simulink model ""  (R2025a)
settings: Solver=FixedStepDiscrete  StartTime=0.0  StopTime=inf  FixedStep=0.001  RelTol=1e-3  EnableMultiTasking=on
PreLoadFcn:
  | frs = FrankaRobotSettings;
libraries: franka_simulink x1
settings Model: SimulationMode=external  ExtModeTrigDuration=10000  Creator=vasi_ko  LastModifiedBy=kvasios
settings SolverCC: AllowMultiTaskInputOutput=on  ConcurrentTasks=on  AlgebraicLoopSolver=TrustRegion  AutoInsertRateTranBlk=on  InsertRTBMode=Never (minimum delay)
settings DataIOCC: LimitDataPoints=on  SaveFormat=Array  ReturnWorkspaceOutputs=off
settings OptimizationCC: DefaultParameterBehavior=Inlined  EnhancedBackFolding=on  PassReuseOutputArgsThreshold=0.0  ZeroExternalMemoryAtStartup=off  ZeroInternalMemoryAtStartup=off  MaxStackSize=200000  OptimizeBlockOrder=speed  DifferentSizesBufferReuse=on  OptimizationCustomize=off
settings DebuggingCC: SolverPrmCheckMsg=warning  ParameterTunabilityLossMsg=error  UnconnectedInputMsg=warning  UnconnectedOutputMsg=warning  UnconnectedLineMsg=warning  SFUnexpectedBacktrackingDiag=warning  SFNoUnconditionalDefaultTransitionDiag=warning  SFExecutionAtInitializationDiag=none  ArithmeticOperatorsInVariantConditions=warning
settings HardwareCC: ProdBitPerLong=64.0  ProdHWDeviceType=Intel->x86-64 (Linux 64)
settings ModelReferenceCC: EnableRefExpFcnMdlSchedulingChecks=on  PropagateSignalLabelsOutOfModel=off
settings SFSimCC: SimUseLocalCustomCode=off  MATLABDynamicMemAlloc=off  CustomCodeUndefinedFunction=UseInterfaceOnly  SimTargetLang=C++  SimDLTargetLibrary=mkl-dnn
settings RTWCC: HardwareBoard=Generic Linux AMD64 Board  RTWVerbose=off  RTWUseLocalCustomCode=off  BuildConfiguration=Faster Runs  TargetLang=C++  GPUComputeCapability=3.5  DLArmComputeVersion=19.05
settings CodeAppCC: ForceParamTrailComments=on  OperatorAnnotations=on
settings GRTTargetCC: ExtModeStaticAlloc=on  ExtModeMexFile=ext_xcp  ExtModeIntrfLevel=Level2 - Open  MultiInstanceErrorCode=Warning  TargetLangStandard=C++14 (ISO)  CodeInterfacePackaging=C++ class  SubcomponentCodeInterfacePackaging=C++ class
settings ConfigComp: CovMetricSettings=dw  CovSaveCumulativeToWorkspaceVar=on  CovSaveSingleToWorkspaceVar=on  CovExternalEMLEnable=off  CovSFcnEnable=off

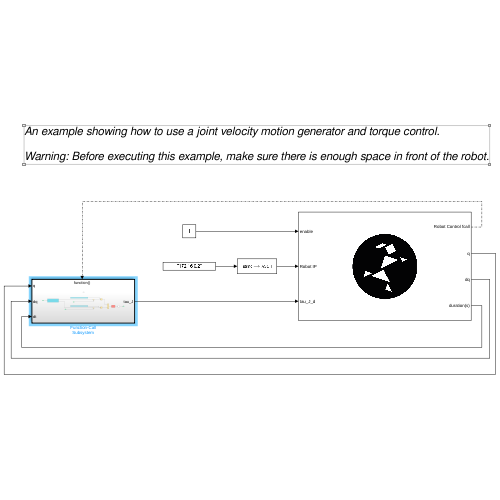
[thumbnail: Simulink's stored preview of the top-level diagram]
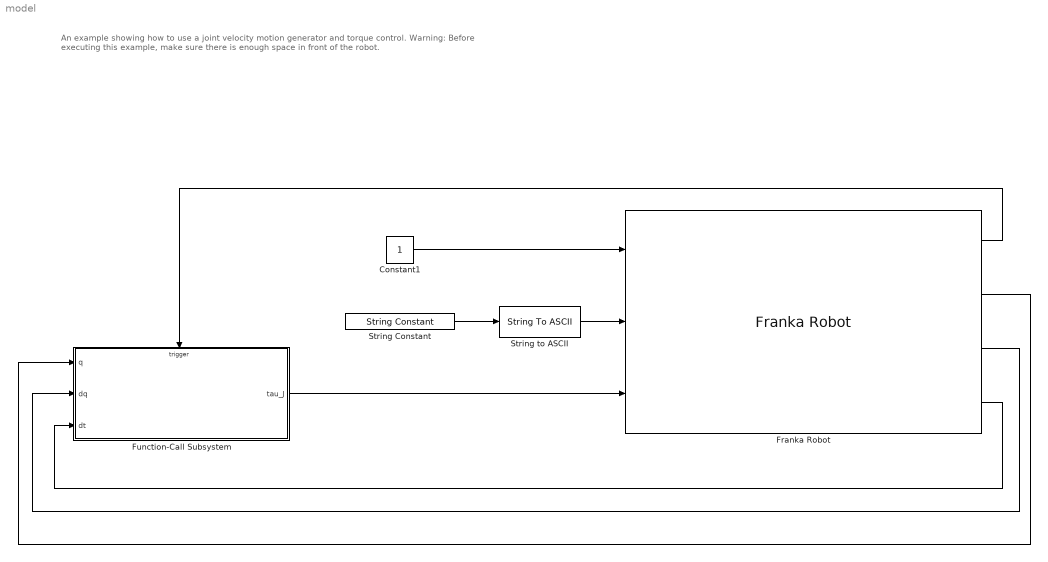
== system model ==
  note: An example showing how to use a joint velocity motion generator and torque control.
      |
      | Warning: Before executing this example, make sure there is enough space in front of the robot.
  Constant1 : Constant
  Franka Robot : franka_simulink/Franka Robot
      settings: SourceProductName=Franka Robotics Simulink Support Package
  Function-Call Subsystem : Subsystem  TreatAsAtomicUnit=on
      settings: RTWSystemCode=Nonreusable function
  String Constant : StringConstant  String="\"172.16.0.2\""
  String to ASCII : StringToASCII  OutputVectorSize=16
  wires:
  Function-Call Subsystem/1(tau_J) -> Franka Robot/3
  Constant1/1 -> Franka Robot/1
  String to ASCII/1 -> Franka Robot/2
  String Constant/1 -> String to ASCII/1
  Franka Robot/4 -> Function-Call Subsystem/3(dt)
  Franka Robot/3 -> Function-Call Subsystem/2(dq)
  Franka Robot/2 -> Function-Call Subsystem/1(q)
  Franka Robot/1 -> Function-Call Subsystem/Trigger

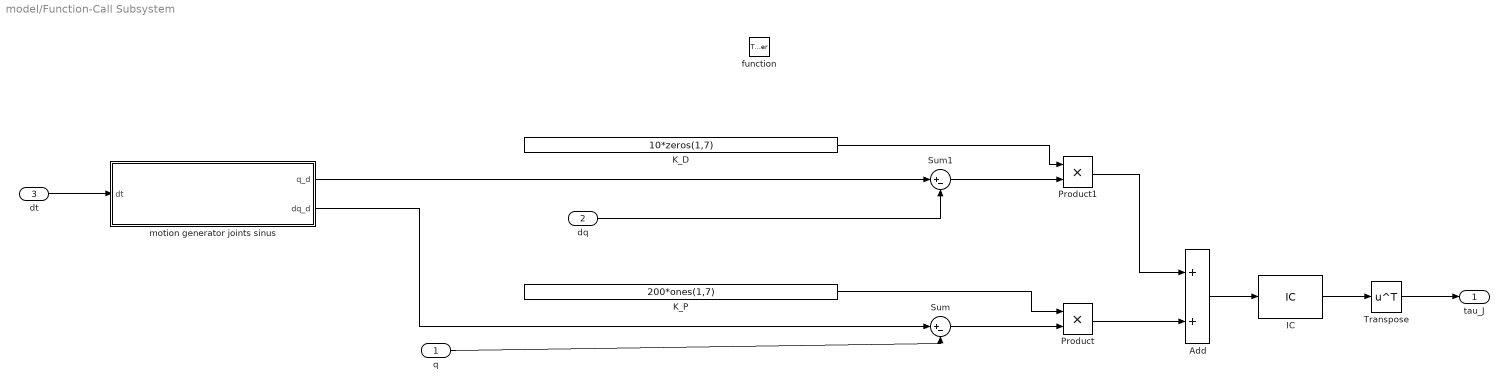
== system model/Function-Call Subsystem ==
  q : Inport
  dq : Inport  Port=2
  dt : Inport  Port=3
  function : TriggerPort  TriggerType=function-call  VariantControl=(inherit)  SampleTime=0.001
  Add : Sum
  IC : InitialCondition  Value=zeros(1,7)
  K_D : Constant  Value=10*zeros(1,7)  VectorParams1D=off  SampleTime=-1
  K_P : Constant  Value=200*ones(1,7)  VectorParams1D=off  SampleTime=-1
  Product : Product
  Product1 : Product
  Sum : Sum  Inputs=|+-
  Sum1 : Sum  Inputs=|+-
  Transpose : Math  Operator=transpose
  motion generator joints sinus : Subsystem
      mask Display:
      | pos = get_param(gcb, 'Position');
      | width = pos(3) - pos(1);
      | x = [0:width];
      | y = sin(x/180*pi);
      | % Parameters 'm' and 'b' must be defined in 'Parameters & Dialog' pane.
      | plot(x,y );
      | 
      | port_label('output',1,'dq_d');
      | port_label('output',2,'q_d');
  tau_J : Outport  VectorParamsAs1DForOutWhenUnconnected=off
  wires:
  IC/1 -> Transpose/1
  Product1/1 -> Add/1
  Sum1/1 -> Product1/2
  dq/1 -> Sum1/2
  Product/1 -> Add/2
  Sum/1 -> Product/2
  Transpose/1 -> tau_J/1
  K_D/1 -> Product1/1
  motion generator joints sinus/1(q_d) -> Sum1/1
  Add/1 -> IC/1
  q/1 -> Sum/2
  K_P/1 -> Product/1
  motion generator joints sinus/2(dq_d) -> Sum/1
  dt/1 -> motion generator joints sinus/1(dt)

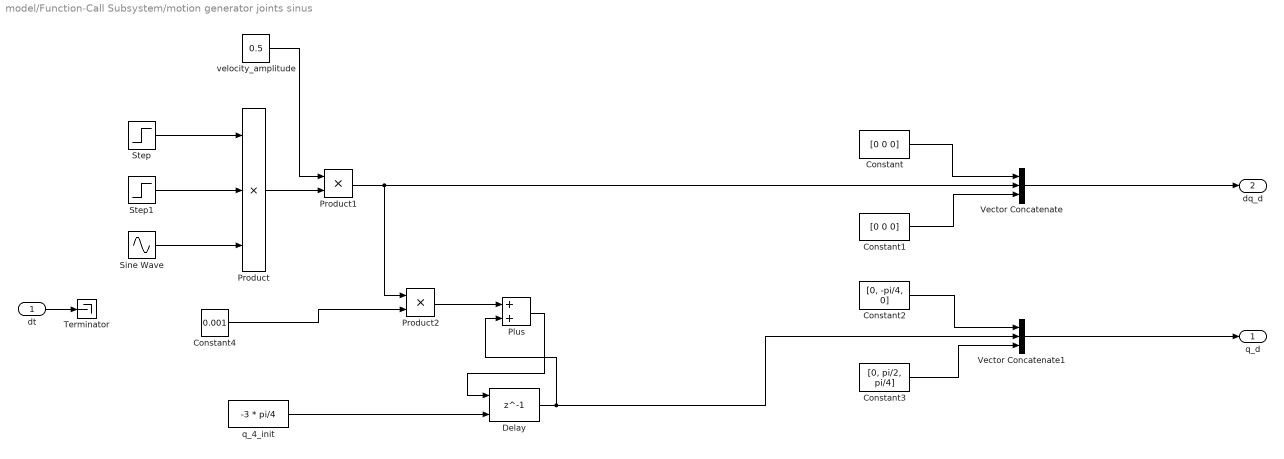
== system model/Function-Call Subsystem/motion generator joints sinus ==
  dt : Inport
  Constant : Constant  Value=[0 0 0]  VectorParams1D=off
  Constant1 : Constant  Value=[0 0 0]  VectorParams1D=off
  Constant2 : Constant  Value=[0, -pi/4, 0]  VectorParams1D=off
  Constant3 : Constant  Value=[0, pi/2, pi/4]  VectorParams1D=off
  Constant4 : Constant  Value=0.001
  Delay : Delay  DelayLength=1  InitialConditionSource=Input port
      settings: InputPortMap=u0,p4
  Plus : Sum
  Product : Product  Inputs=3
  Product1 : Product
  Product2 : Product
  Sine Wave : Sin  Frequency=pi  Phase=pi
  Step : Step
  Step1 : Step  Time=7  Before=1  After=0
  Terminator : Terminator
  Vector Concatenate : Concatenate  NumInputs=3
  Vector Concatenate1 : Concatenate  NumInputs=3
  q_4_init : Constant  Value=-3 * pi/4  VectorParams1D=off
  velocity_amplitude : Constant  Value=0.5  VectorParams1D=off
  q_d : Outport  VectorParamsAs1DForOutWhenUnconnected=off
  dq_d : Outport  Port=2  VectorParamsAs1DForOutWhenUnconnected=off
  wires:
  Constant1/1 -> Vector Concatenate/3
  Constant/1 -> Vector Concatenate/1
  Product/1 -> Product1/2
  Sine Wave/1 -> Product/3
  Step/1 -> Product/1
  velocity_amplitude/1 -> Product1/1
  Product1/1 -> Vector Concatenate/2, Product2/1
  Vector Concatenate/1 -> dq_d/1
  Constant3/1 -> Vector Concatenate1/3
  Constant2/1 -> Vector Concatenate1/1
  Vector Concatenate1/1 -> q_d/1
  q_4_init/1 -> Delay/2
  Step1/1 -> Product/2
  Delay/1 -> Vector Concatenate1/2, Plus/2
  Plus/1 -> Delay/1
  Product2/1 -> Plus/1
  dt/1 -> Terminator/1
  Constant4/1 -> Product2/2
